simulink model "Task_7"  (R2022b)
settings: Solver=VariableStepAuto  StartTime=0.0  StopTime=10.0  RelTol=1e-3
settings Model: Creator=Abanob_Sameh  LastModifiedBy=Abanob_Sameh

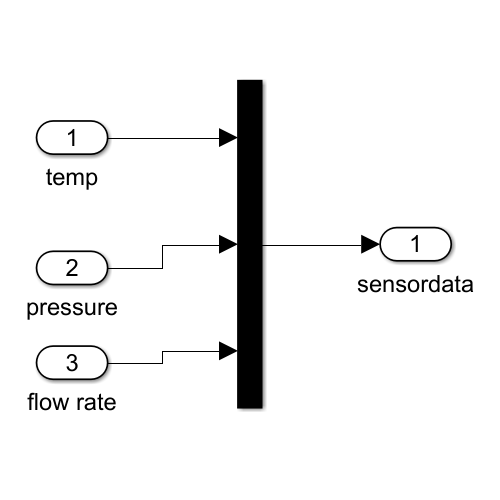
[thumbnail: Simulink's stored preview of the top-level diagram]
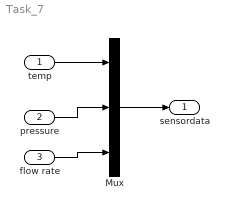
== system Task_7 ==
  temp : Inport
  pressure : Inport  Port=2
  flow rate : Inport  Port=3
  Mux : Mux  Inputs=3
  sensordata : Outport
  wires:
  temp/1 -> Mux/1
  pressure/1 -> Mux/2
  flow rate/1 -> Mux/3
  Mux/1 -> sensordata/1
